simulink model "sim_test_stateFB"  (R2016a)
settings: Solver=ode3  StartTime=0.0  StopTime=Tsim  FixedStep=Ts  RelTol=1e-3
undefined symbols (not defined in the file): Aof, Bof, Cof, dist, Dof, K, P1, ref, Tdist, Tref, Tutest, utest, x0
settings Model: Creator=Matti  LastModifiedBy=Matti

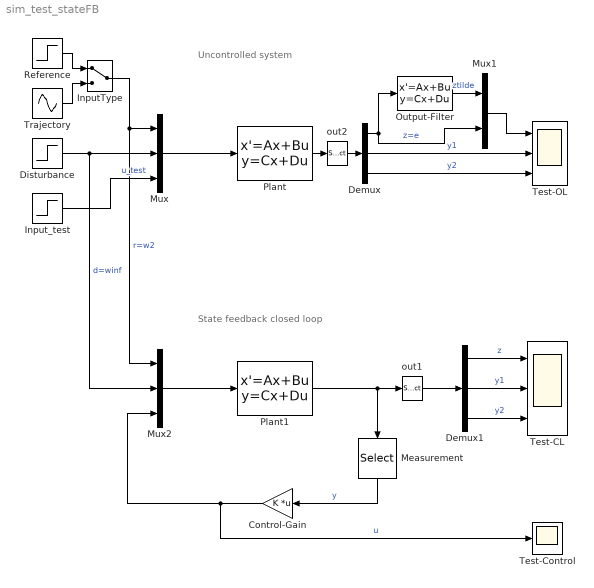
== system sim_test_stateFB ==
  note: State feedback closed loop
  note: Uncontrolled system
  Control-Gain : Gain  Gain=K  Multiplication=Matrix(K*u)
  Demux : Demux  Outputs=3
  Demux1 : Demux  Outputs=3
  Disturbance : Step  Time=Tdist  After=dist  SampleTime=0
  InputType : ManualSwitch
  Input_test : Step  Time=Tutest  After=utest  SampleTime=0
  Measurement : Selector  InputPortWidth=4  IndexOptions=Index vector (dialog)  Indices=[3 4]  OutputSizes=1
  Mux : Mux  Inputs=3
  Mux1 : Mux  Inputs=2
  Mux2 : Mux  Inputs=3
  Output-Filter : StateSpace  A=Aof  B=Bof  C=Cof  D=Dof  X0=0
  Plant : StateSpace  A=P1.A  B=P1.B  C=P1.C  D=P1.D  X0=x0
  Plant1 : StateSpace  A=P1.A  B=P1.B  C=P1.C  D=P1.D  X0=x0
  Reference : Step  Time=Tref  After=ref  SampleTime=0
  Test-CL : Scope  NumInputPorts=3
  Test-Control : Scope
  Test-OL : Scope  NumInputPorts=3
  Trajectory : Sin  Frequency=0.5  SampleTime=0
  out1 : Selector  InputPortWidth=4  IndexOptions=Index vector (dialog)  Indices=[1 3 4]  OutputSizes=1
  out2 : Selector  InputPortWidth=4  IndexOptions=Index vector (dialog)  Indices=[1 3 4]  OutputSizes=1
  wires:
  Mux/1 -> Plant/1
  Disturbance/1 -> Mux2/2, Mux/2  "d=winf"
  Input_test/1 -> Mux/3  "u_test"
  Demux/1 -> Output-Filter/1, Mux1/2  "z=e"
  Demux/2 -> Test-OL/2  "y1"
  Demux/3 -> Test-OL/3  "y2"
  Output-Filter/1 -> Mux1/1  "ztilde"
  Measurement/1 -> Control-Gain/1  "y"
  Plant1/1 -> Measurement/1, out1/1
  Control-Gain/1 -> Test-Control/1, Mux2/3  "u"
  Demux1/3 -> Test-CL/3  "y2"
  Demux1/2 -> Test-CL/2  "y1"
  Mux2/1 -> Plant1/1
  Reference/1 -> InputType/1
  InputType/1 -> Mux/1, Mux2/1  "r=w2"
  Trajectory/1 -> InputType/2
  Mux1/1 -> Test-OL/1
  Demux1/1 -> Test-CL/1  "z"
  out1/1 -> Demux1/1
  out2/1 -> Demux/1
  Plant/1 -> out2/1
